simulink model "jiashangzhouqihanshude"  (Simulink 7.4)
settings: Solver=ode45  StartTime=0.0  StopTime=5  RelTol=1e-3
libraries: simulink x1
settings Model: Creator=admini  LastModifiedBy=admini

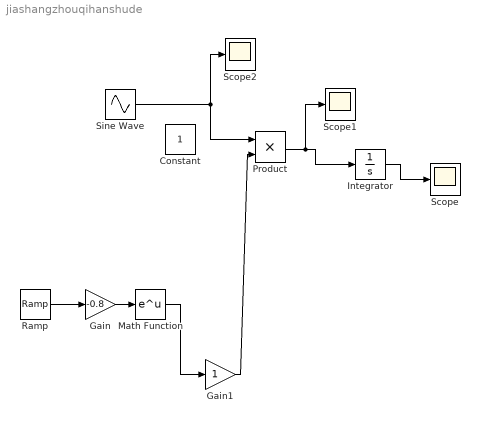
== system jiashangzhouqihanshude ==
  Constant : Constant  OutDataType=fixdt(1, 16)  OutScaling=2^0
  Gain : Gain  Gain=-0.8  ParameterDataType=fixdt(1, 16)  ParameterScaling=2^0  OutDataType=fixdt(1, 16)  OutScaling=2^0
  Gain1 : Gain  ParameterDataType=fixdt(1, 16)  ParameterScaling=2^0  OutDataType=fixdt(1, 16)  OutScaling=2^0
  Integrator : Integrator
  Math Function : Math  OutDataType=fixdt(1, 16)  OutScaling=2^0  SaturateOnIntegerOverflow=on
  Product : Product  OutDataType=fixdt(1, 16)  OutScaling=2^0  RndMeth=Zero
  Ramp : simulink/Sources/Ramp  SystemSampleTime=-1  slope=1  start=0  X0=0
  Scope : Scope
      settings: TimeRange=100  YMin=0  YMax=0.7000000000000001
  Scope1 : Scope
  Scope2 : Scope
      settings: SaveName=ScopeData2
  Sine Wave : Sin  Amplitude=0.3  Bias=0.6  Frequency=2  Phase=0  Samples=2  SampleTime=0  Offset=0
  wires:
  Gain/1 -> Math Function/1
  Integrator/1 -> Scope/1
  Sine Wave/1 -> Scope2/1, Product/1
  Product/1 -> Integrator/1, Scope1/1
  Math Function/1 -> Gain1/1
  Gain1/1 -> Product/2
  Ramp/1 -> Gain/1
